simulink model "bike_model_position_pid_alone"  (R2018b)
settings: Solver=FixedStepAuto  StartTime=0.0  StopTime=200  FixedStep=0.04  RelTol=1e-3
values from neighbouring files (symbols this model uses):
  initial_x = x_ini_diff    (= 0)    [paths.m]
  initial_y = y_ini_diff    (= 0)    [paths.m]
  Ts = 0.04    [configuration.m]    (also in configuration_boxMovedCenter.m; configuration_pidTuning.m; positionEstimation.m)
libraries: simulink x2, dspsigops x1
settings Model: Creator=maximef  LastModifiedBy=maximef

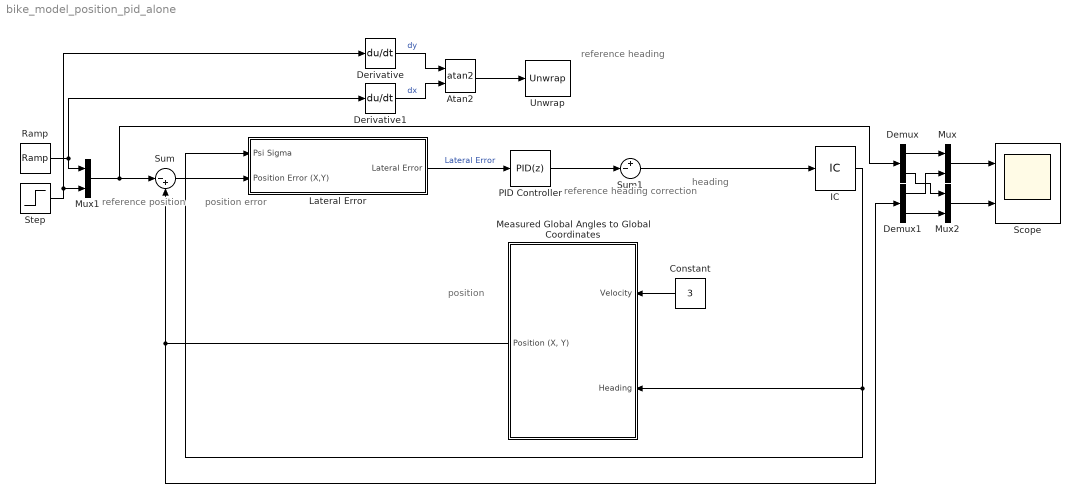
== system bike_model_position_pid_alone ==
  note: heading
  note: reference
      | position
  note: position
  note: reference
      | heading
      | correction
  note: reference
      | heading
  note: position
      | error
  Atan2 : Trigonometry  Operator=atan2
  Constant : Constant  Value=3
  Demux : Demux  Outputs=2
  Demux1 : Demux  Outputs=2
  Derivative : Derivative
  Derivative1 : Derivative
  IC : InitialCondition  Value=0
  Lateral Error : Subsystem  SystemSampleTime=Ts
  Measured Global Angles to Global Coordinates : Subsystem
  Mux : Mux  Inputs=2
  Mux1 : Mux  Inputs=2
  Mux2 : Mux  Inputs=2
  PID Controller : simulink/Continuous/PID Controller  Controller=PID  Form=Parallel  TimeDomain=Discrete-time  SampleTime=0.04  IntegratorMethod=Forward Euler  FilterMethod=Forward Euler  ControllerParametersSource=internal  P=0.4  I=0  D=0  UseFilter=off  N=1.75931167589302  TunerSelectOption=Transfer Function Based (PID Tuner App)  InitialConditionSource=internal  InitialConditionForIntegrator=0  InitialConditionForFilter=0  DifferentiatorICPrevScaledInput=0  ExternalReset=none  TrackingMode=off  Kt=1  LimitOutput=off  UpperSaturationLimit=inf  LowerSaturationLimit=-inf  LinearizeAsGain=on  AntiWindupMode=none  Kb=1  POutMin=[]  POutMax=[]  IOutMin=[]  IOutMax=[]  DOutMin=[]  DOutMax=[]  NOutMin=[]  NOutMax=[]  SumOutMin=[]  SumOutMax=[]  SaturationOutMin=[]  SaturationOutMax=[]  PParamMin=[]  PParamMax=[]  IParamMin=[]  IParamMax=[]  DParamMin=[]  DParamMax=[]  NParamMin=[]  NParamMax=[]  KbParamMin=[]  KbParamMax=[]  KtParamMin=[]  KtParamMax=[]  KbOutMin=[]  KbOutMax=[]  KtOutMin=[]  KtOutMax=[]  IntegratorOutMin=[]  IntegratorOutMax=[]  FilterOutMin=[]  FilterOutMax=[]  SumI1OutMin=[]  SumI1OutMax=[]  SumI2OutMin=[]  SumI2OutMax=[]  SumI3OutMin=[]  SumI3OutMax=[]  SumI4OutMin=[]  SumI4OutMax=[]  SumDOutMin=[]  SumDOutMax=[]  DifferentiatorOutMin=[]  DifferentiatorOutMax=[]  FilterDiffOutCoefMin=[]  FilterDiffOutCoefMax=[]  ReciprocalOutMin=[]  ReciprocalOutMax=[]  SumDenOutMin=[]  SumDenOutMax=[]  SumNumOutMin=[]  SumNumOutMax=[]  DivideOutMin=[]  DivideOutMax=[]  IntegratorContinuousStateAttributes=''  IntegratorStateMustResolveToSignalObject=off  IntegratorRTWStateStorageClass=Auto  FilterContinuousStateAttributes=''  FilterStateMustResolveToSignalObject=off  FilterRTWStateStorageClass=Auto  ParallelPVariant=InternalParameters  IdealPVariant=Disabled  IVariant=InternalParameters  DVariant=InternalParameters  IntegratorVariant=Discrete  SatVariant=Disabled  AWVariant=Passthrough  PCopyVariant=Disabled  TRVariant=Disabled  FdbkBlocksVariant=Forward  IdealPFdbkVariant=Disabled  SatFdbkVariant=Disabled  DerivativeFilterVariant=Differentiator  NVariant=Passthrough  NCopyVariant=Disabled_SignalSpec  FilterICVariant=InternalICsDifferentiator  IntegratorICVariant=InternalICs  ExternalResetVariant=Disabled  TRSumVariant=Passthrough  SumFdbkVariant=Disabled  SumVariant=Sum_PID
  Ramp : simulink/Sources/Ramp  slope=3  start=0  InitialOutput=0
  Scope : Scope  NumInputPorts=2
  Step : Step  Time=5  After=0.1  SampleTime=0
  Sum : Sum  Inputs=|-+
  Sum1 : Sum  Inputs=+-|
  Unwrap : dspsigops/Unwrap  tol=pi  InputProcessing=Columns as channels (frame based)  running=off
  wires:
  Step/1 -> Derivative/1, Mux1/2
  Mux1/1 -> Demux/1, Sum/1
  Ramp/1 -> Mux1/1, Derivative1/1
  Constant/1 -> Measured Global Angles to Global Coordinates/1(Velocity)
  Derivative/1 -> Atan2/1  "dy"
  Atan2/1 -> Unwrap/1
  Lateral Error/1(Lateral Error) -> PID Controller/1  "Lateral Error"
  Demux/2 -> Mux2/1
  Mux2/1 -> Scope/2
  Demux1/1 -> Mux/2
  Sum/1 -> Lateral Error/2(Position Error (X,Y))
  Mux/1 -> Scope/1
  Demux/1 -> Mux/1
  Derivative1/1 -> Atan2/2  "dx"
  Demux1/2 -> Mux2/2
  Measured Global Angles to Global Coordinates/1("Position (X, Y)") -> Sum/2, Demux1/1
  Sum1/1 -> IC/1
  ? -> Sum1/1
  IC/1 -> Lateral Error/1(Psi Sigma), Measured Global Angles to Global Coordinates/2(Heading)
  PID Controller/1 -> Sum1/2

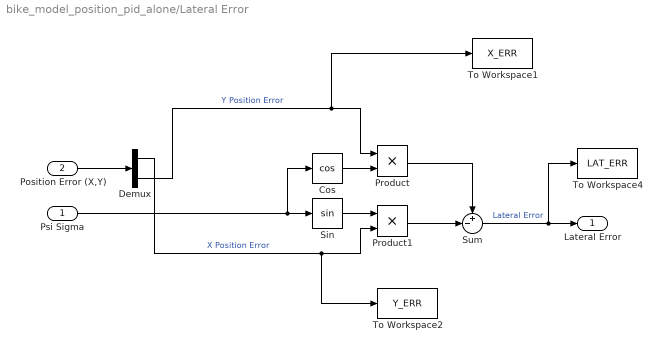
== system bike_model_position_pid_alone/Lateral Error ==
  Psi Sigma : Inport
  Position Error (X,Y) : Inport  Port=2
  Cos : Trigonometry  Operator=cos
  Demux : Demux  Outputs=2
  Product : Product
  Product1 : Product
  Sin : Trigonometry
  Sum : Sum  Inputs=+-|
  To Workspace1 : ToWorkspace  VariableName=X_ERR  SaveFormat=Timeseries  SampleTime=Ts
  To Workspace2 : ToWorkspace  VariableName=Y_ERR  SaveFormat=Timeseries  SampleTime=Ts
  To Workspace4 : ToWorkspace  VariableName=LAT_ERR  SaveFormat=Timeseries  SampleTime=Ts
  Lateral Error : Outport
  wires:
  Cos/1 -> Product/2
  Sin/1 -> Product1/1
  Psi Sigma/1 -> Cos/1, Sin/1
  Product/1 -> Sum/1
  Sum/1 -> To Workspace4/1, Lateral Error/1  "Lateral Error"
  Demux/1 -> To Workspace2/1, Product1/2  "X Position Error"
  Demux/2 -> To Workspace1/1, Product/1  "Y Position Error"
  Position Error (X,Y)/1 -> Demux/1
  Product1/1 -> Sum/2

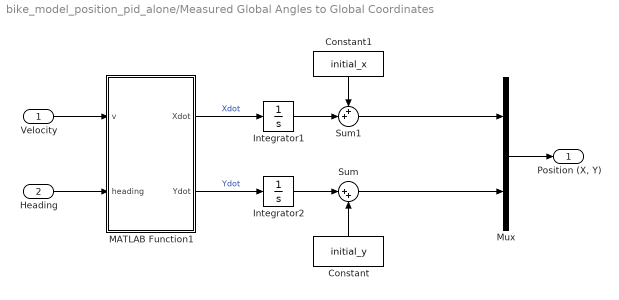
== system bike_model_position_pid_alone/Measured Global Angles to Global Coordinates ==
  Velocity : Inport
  Heading : Inport  Port=2
  Constant : Constant  Value=initial_y
  Constant1 : Constant  Value=initial_x
  Integrator1 : Integrator
  Integrator2 : Integrator
  MATLAB Function1 : MATLAB Function  TreatAsAtomicUnit=on
  Mux : Mux  Inputs=2
  Sum : Sum  Inputs=|++
  Sum1 : Sum  Inputs=++|
  "Position (X, Y)" : Outport
  wires:
  MATLAB Function1/2(Ydot) -> Integrator2/1  "Ydot"
  MATLAB Function1/1(Xdot) -> Integrator1/1  "Xdot"
  Heading/1 -> MATLAB Function1/2(heading)
  Velocity/1 -> MATLAB Function1/1(v)
  Integrator2/1 -> Sum/1
  Constant/1 -> Sum/2
  Sum/1 -> Mux/2
  Integrator1/1 -> Sum1/2
  Sum1/1 -> Mux/1
  Constant1/1 -> Sum1/1
  Mux/1 -> "Position (X, Y)"/1

== matlab function bike_model_position_pid_alone/Measured Global Angles to Global Coordinates/MATLAB Function1 ==
  data: v input; heading input; Xdot output; Ydot output
function [Xdot, Ydot]  = fcn(v, heading)

Xdot = v * cos(heading);
Ydot = v * sin(heading);
